simulink model "aufgabe4_sim"  (R2016b)
settings: Solver=VariableStepAuto  StartTime=0.0  StopTime=14  RelTol=1e-3
values from neighbouring files (symbols this model uses):
  A = double([0, 1, -1; -3411/62, -54163/28520, 1/1240;      6822/325, 1/3250, 54117/74750 - (7*1130385^(1/2))/7475])    [aufgabe1.m]    (also in aufgabe2.m; aufgabe3.m; aufgabe4.m; aufgabe5.m)
  bd = double([0; 0; -400/13])    [aufgabe1.m]    (also in aufgabe2.m; aufgabe3.m; aufgabe4.m; aufgabe5.m)
  bu = double([0; 12500/713; 0])    [aufgabe1.m]    (also in aufgabe2.m; aufgabe3.m; aufgabe4.m; aufgabe5.m)
  ct = [0 0 1]    [aufgabe1.m]    (also in aufgabe2.m; aufgabe3.m; aufgabe4.m; aufgabe5.m)
  kI = ke(4)    [aufgabe3.m]    (also in aufgabe4.m = 0.0065; aufgabe5.m = 0.0065)
  kP = 1/(ct*inv(eye(3)-phi)*gamma)    [aufgabe3.m]    (also in aufgabe4.m = 0.1488; aufgabe5.m = 0.1488)
  kx = kP*ct+ke(1:3)    [aufgabe3.m]    (also in aufgabe4.m = [-0.6050   -0.7335    0.3827]; aufgabe5.m = [-0.6050   -0.7335    0.3827])
  Ta = 10e-03    (= 0.01)    [aufgabe1.m]    (also in aufgabe2.m; aufgabe3.m; aufgabe4.m; aufgabe5.m)
  u_GSM_r = 5.6    [aufgabe2.m]    (also in aufgabe3.m; aufgabe4.m; aufgabe6.m; aufgabe7.m)
  w_P_r = x_R(4)    [aufgabe2.m]    (also in aufgabe3.m = -(R_GSM*d_vP + R_GSM*d_vGSM - (k_GSM^4 + R_GSM^2*d_vP^2 +   ; aufgabe4.m = -(R_GSM*d_vP + R_GSM*d_vGSM - (k_GSM^4 + R_GSM^2*d_vP^2 +   ; aufgabe6.m = -(R_GSM*d_vP + R_GSM*d_vGSM - (k_GSM^4 + R_GSM^2*d_vP^2 +   ; aufgabe7.m = -(R_GSM*d_vP + R_GSM*d_vGSM - (k_GSM^4 + R_GSM^2*d_vP^2 +   )
  x_r = [i_GSM_r; phi_GSMP_r; w_GSM_r; w_P_r]    [aufgabe3.m]    (also in aufgabe4.m; aufgabe6.m; aufgabe7.m)
undefined symbols (not defined in the file): c_GSMP, d_cGSM, d_cP, d_GSMP, d_qP, d_vGSM, d_vP, i_GSM_0, J_GSM, J_P, k_GSM, L_GSM, phi_GSMP_0, R_GSM, w_GSM_0, w_P_0
libraries: cstblocks x1, simulink x1
settings Model: Creator=M  LastModifiedBy=M

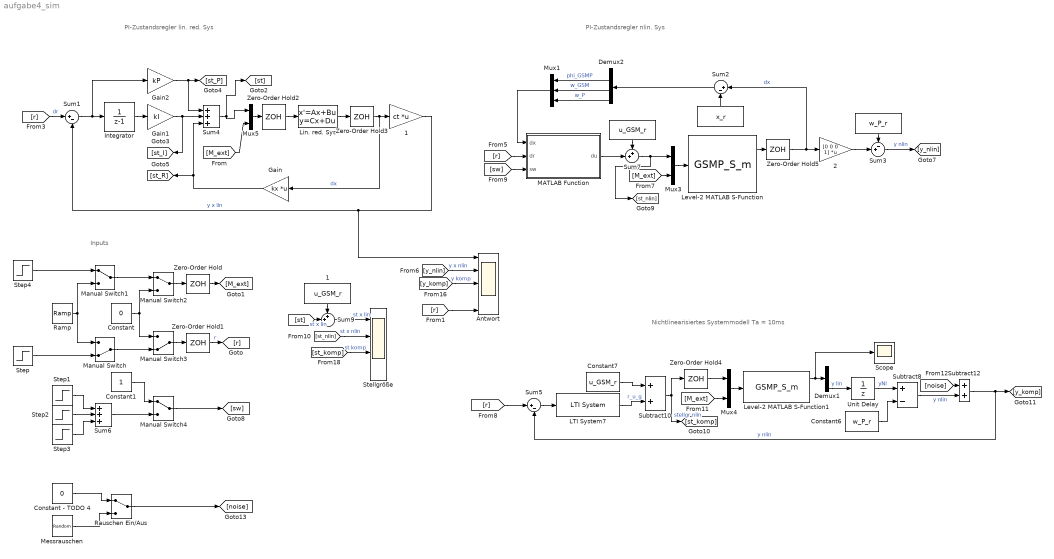
== system aufgabe4_sim ==
  note: Inputs
  note: PI-Zustandsregler lin. red. Sys
  note: PI-Zustandsregler nlin. Sys
  note: Nichtlinearisiertes Systemmodell Ta = 10ms
  " " : Constant  Value=u_GSM_r
  " " : Constant  Value=w_P_r
  " 1" : Constant  Value=u_GSM_r
  " " : Constant  Value=x_r
  "   1" : Gain  Gain=ct  Multiplication=Matrix(K*u)
  "   2" : Gain  Gain=[0 0 0 1]  Multiplication=Matrix(K*u)
  Antwort : Scope  NumInputPorts=5
  Constant : Constant  Value=0
  Constant - TODO 4 : Constant  Value=0
  Constant1 : Constant
  Constant6 : Constant  Value=w_P_r
  Constant7 : Constant  Value=u_GSM_r
  Demux1 : Demux
  Demux2 : Demux
  Gain : Gain  Gain=kx  Multiplication=Matrix(K*u)  SampleTime=Ta
  Gain1 : Gain  Gain=kI
  Gain2 : Gain  Gain=kP
  Integrator : DiscreteTransferFcn  Denominator=[1 -1]  SampleTime=Ta
  LTI System7 : cstblocks/LTI System  sys=R_komp  IC=[]
  Level-2 MATLAB S-Function : M-S-Function  FunctionName=GSMP_S_m  Parameters=L_GSM, R_GSM, k_GSM, J_GSM, d_cGSM, d_vGSM, J_P, d_cP, d_vP, d_qP, c_GSMP, d_GSMP, i_GSM_0, phi_GSMP_0, w_GSM_0, w_P_0  mask{L_GSM=L_GSM, R_GSM=R_GSM, k_GSM=k_GSM, J_GSM=J_GSM, d_cGSM=d_cGSM, d_vGSM=d_vGSM, J_P=J_P, d_cP=d_cP, d_vP=d_vP, d_qP=d_qP, c_GSMP=c_GSMP, d_GSMP=d_GSMP, i_GSM_0=i_GSM_0, phi_GSMP_0=phi_GSMP_0, w_GSM_0=w_GSM_0, w_P_0=w_P_0}
      mask prompts: i_GSM_0 "i_GSM"; phi_GSMP_0 "phi_GSMP"; w_GSM_0 "w_GSM"; w_P_0 "w_P"
      mask DialogControl Container3 Prompt: Anfangszustände
  Level-2 MATLAB S-Function1 : M-S-Function  FunctionName=GSMP_S_m  Parameters=L_GSM, R_GSM, k_GSM, J_GSM, d_cGSM, d_vGSM, J_P, d_cP, d_vP, d_qP, c_GSMP, d_GSMP, i_GSM_0, phi_GSMP_0, w_GSM_0, w_P_0  mask{L_GSM=L_GSM, R_GSM=R_GSM, k_GSM=k_GSM, J_GSM=J_GSM, d_cGSM=d_cGSM, d_vGSM=d_vGSM, J_P=J_P, d_cP=d_cP, d_vP=d_vP, d_qP=d_qP, c_GSMP=c_GSMP, d_GSMP=d_GSMP, i_GSM_0=i_GSM_0, phi_GSMP_0=phi_GSMP_0, w_GSM_0=w_GSM_0, w_P_0=w_P_0}
      mask prompts: i_GSM_0 "i_GSM"; phi_GSMP_0 "phi_GSMP"; w_GSM_0 "w_GSM"; w_P_0 "w_P"
      mask DialogControl Container3 Prompt: Anfangszustände
  Lin. red. Sys : StateSpace  A=A  B=[bu bd]  C=eye(3)  D=[0 0; 0 0; 0 0]  X0=[0,0,0]
  MATLAB Function : MATLAB Function  TreatAsAtomicUnit=on  SystemSampleTime=Ta
  Manual Switch : ManualSwitch  CurrentSetting=0
  Manual Switch1 : ManualSwitch
  Manual Switch2 : ManualSwitch
  Manual Switch3 : ManualSwitch  CurrentSetting=0
  Manual Switch4 : ManualSwitch
  Messrauschen : UniformRandomNumber  Minimum=-5e-2  Maximum=5e-2  SampleTime=1e-3
  Mux1 : Mux  Inputs=3
  Mux3 : Mux  Inputs=2
  Mux4 : Mux  Inputs=2
  Mux5 : Mux  Inputs=2
  Ramp : simulink/Sources/Ramp  slope=1  start=1  X0=0
  Rauschen Ein/Aus : ManualSwitch
  Scope : Scope
  Stellgröße : Scope  NumInputPorts=4
  Step : Step  After=20  SampleTime=0
  Step1 : Step  SampleTime=0
  Step2 : Step  Time=5  After=-1  SampleTime=0
  Step3 : Step  Time=10  SampleTime=0
  Step4 : Step  Time=5  After=-0.5  SampleTime=0
  Subtract10 : Sum
  Subtract12 : Sum
  Subtract8 : Sum  Inputs=+-
  Sum1 : Sum  Inputs=|+-
  Sum2 : Sum  Inputs=|+-
  Sum3 : Sum  Inputs=-+|
  Sum4 : Sum  Inputs=+++
  Sum5 : Sum  Inputs=|+-
  Sum6 : Sum  Inputs=+++
  Sum7 : Sum  Inputs=++|
  Sum9 : Sum  Inputs=++|
  Unit Delay : UnitDelay  InitialCondition=w_P_r  SampleTime=Ta
  Zero-Order Hold : ZeroOrderHold  SampleTime=-1
  Zero-Order Hold1 : ZeroOrderHold  SampleTime=-1
  Zero-Order Hold{2..5} (4 alike) : ZeroOrderHold  SampleTime=Ta
  wires:
  Manual Switch1/1 -> Manual Switch2/1
  Constant/1 -> Manual Switch3/1, Manual Switch2/2
  Manual Switch2/1 -> Zero-Order Hold/1
  Manual Switch3/1 -> Zero-Order Hold1/1
  Manual Switch/1 -> Manual Switch3/2
  Ramp/1 -> Manual Switch/1, Manual Switch1/2
  Step/1 -> Manual Switch/2
  Zero-Order Hold1/1 -> [r]  "r"
  Zero-Order Hold/1 -> [M_ext]
  Zero-Order Hold2/1 -> Lin. red. Sys/1
  Sum1/1 -> Gain2/1, Integrator/1
  Gain1/1 -> [st_I], Sum4/2
  Sum4/1 -> Mux5/1, [st]
  Gain/1 -> Sum4/3, [st_R]
  Lin. red. Sys/1 -> Zero-Order Hold3/1
  Zero-Order Hold3/1 -> Gain/1, "   1"/1  "dx"
  [r] -> Antwort/5
  "   1"/1 -> Sum1/2, Antwort/1  "y x lin"
  Integrator/1 -> Gain1/1
  Gain2/1 -> [st_P], Sum4/1
  [r] -> Sum1/1  "dr"
  [r] -> MATLAB Function/2(dr)
  [sw] -> MATLAB Function/3(sw)
  Mux3/1 -> Level-2 MATLAB S-Function/1
  [M_ext] -> Mux3/2
  Zero-Order Hold5/1 -> "   2"/1, Sum2/1  "dx"
  MATLAB Function/1(du) -> Sum7/2
  Sum7/1 -> [st_nlin], Mux3/1
  Demux2/2 -> Mux1/1  "phi_GSMP"
  Demux2/3 -> Mux1/2  "w_GSM"
  Demux2/4 -> Mux1/3  "w_P"
  Sum2/1 -> Demux2/1
  Mux1/1 -> MATLAB Function/1(dx)
  Level-2 MATLAB S-Function/1 -> Zero-Order Hold5/1
  "   2"/1 -> Sum3/2
  Sum3/1 -> [y_nlin]  "y nlin"
  Step1/1 -> Sum6/1
  Step2/1 -> Sum6/2
  Step3/1 -> Sum6/3
  Sum6/1 -> Manual Switch4/2
  Manual Switch4/1 -> [sw]
  Constant1/1 -> Manual Switch4/1
  [y_nlin] -> Antwort/2  "y x nlin"
  " "/1 -> Sum7/1
  " "/1 -> Sum3/1
  " "/1 -> Sum2/2
  Sum5/1 -> LTI System7/1
  [r] -> Sum5/1
  Demux1/4 -> Unit Delay/1  "y lin"
  Subtract10/1 -> [st_komp], Zero-Order Hold4/1  "stellgr nlin"
  Level-2 MATLAB S-Function1/1 -> Scope/1, Demux1/1
  Mux4/1 -> Level-2 MATLAB S-Function1/1
  Unit Delay/1 -> Subtract8/1  "yNl"
  Zero-Order Hold4/1 -> Mux4/1
  Constant7/1 -> Subtract10/1
  Constant6/1 -> Subtract8/2
  [M_ext] -> Mux4/2
  LTI System7/1 -> Subtract10/2  "r_u_g"
  [noise] -> Subtract12/1
  Subtract8/1 -> Subtract12/2  "y nlin"
  Subtract12/1 -> [y_komp], Sum5/2  "y nlin"
  Messrauschen/1 -> Rauschen Ein/Aus/2
  Constant - TODO 4/1 -> Rauschen Ein/Aus/1
  Rauschen Ein/Aus/1 -> [noise]
  [y_komp] -> Antwort/3  "y komp"
  [st_nlin] -> Stellgröße/2  "st x nlin"
  [st_komp] -> Stellgröße/3  "st komp"
  [st] -> Sum9/2  "st x lin"
  " 1"/1 -> Sum9/1
  Sum9/1 -> Stellgröße/1  "st x lin"
  Step4/1 -> Manual Switch1/1
  Mux5/1 -> Zero-Order Hold2/1
  [M_ext] -> Mux5/2

== matlab function aufgabe4_sim/MATLAB Function ==
  settings: updateMethod=DISCRETE  sampleTime=0.01
  data: dx input; du output; dr input; sw input; parZR parameter
function du = fcn(dx, dr, sw, parZR)

% Zustand
persistent xI;
if(isempty(xI))
    xI = 0;
end

if (sw~=0)
    yk = parZR.c_z*dx;
    du = [parZR.kx parZR.kI]*[dx; xI] + parZR.kp*(dr - yk);
    
    % xI k+1 berechnen
    xI = xI + (dr - yk);
else
    du = 0;
    xI = 0;
end
